simulink model "motorControlSim"  (R2021a)
settings: Solver=VariableStepAuto  StartTime=0.0  StopTime=10  RelTol=1e-3
libraries: fl_lib x9, nesl_utility x9, mcbcontrolslib x8, pid_lib x5, ee_lib x3
settings Model: Creator=Maxim  LastModifiedBy=Max

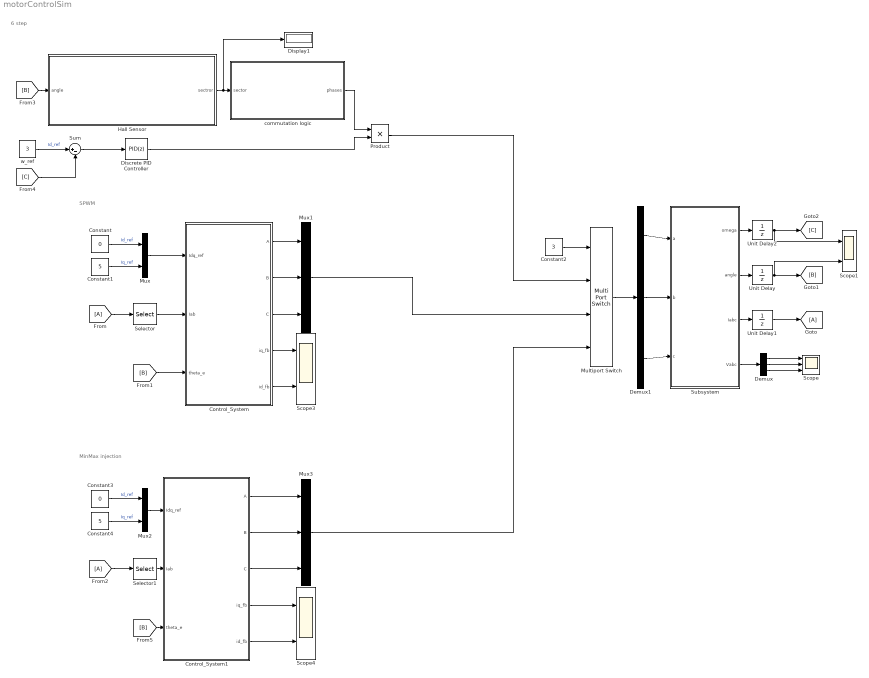
== system motorControlSim ==
  note: 6 step
  note: SPWM
  note: MinMax injection
  Constant : Constant  Value=0  OutDataTypeStr=double
  Constant1 : Constant  Value=5  OutDataTypeStr=double
  Constant2 : Constant  Value=3
  Constant3 : Constant  Value=0  OutDataTypeStr=double
  Constant4 : Constant  Value=5  OutDataTypeStr=double
  Control_System : Subsystem
  Control_System1 : Subsystem
  Demux : Demux  Outputs=3
  Demux1 : Demux  Outputs=3
  Discrete PID Controller : pid_lib/PID Controller  Controller=PID  Form=Parallel  TimeDomain=Discrete-time  UseExternalTs=off  SampleTime=-1  IntegratorMethod=Forward Euler  FilterMethod=Forward Euler  ControllerParametersSource=internal  P=1  I=0.5  D=0  UseFilter=on  N=100  TunerSelectOption=Transfer Function Based (PID Tuner App)  InitialConditionSource=internal  InitialConditionForIntegrator=0  InitialConditionForFilter=0  DifferentiatorICPrevScaledInput=0  ExternalReset=none  TrackingMode=off  Kt=1  LimitOutput=off  SatLimitsSource=internal  UpperSaturationLimit=1  LowerSaturationLimit=0  LinearizeAsGain=off  AntiWindupMode=back-calculation  Kb=1  POutMin=[]  POutMax=[]  IOutMin=[]  IOutMax=[]  DOutMin=[]  DOutMax=[]  NOutMin=[]  NOutMax=[]  SumOutMin=[]  SumOutMax=[]  SaturationOutMin=[]  SaturationOutMax=[]  PParamMin=[]  PParamMax=[]  IParamMin=[]  IParamMax=[]  DParamMin=[]  DParamMax=[]  NParamMin=[]  NParamMax=[]  KbParamMin=[]  KbParamMax=[]  KtParamMin=[]  KtParamMax=[]  KbOutMin=[]  KbOutMax=[]  KtOutMin=[]  KtOutMax=[]  IntegratorOutMin=[]  IntegratorOutMax=[]  FilterOutMin=[]  FilterOutMax=[]  SumI1OutMin=[]  SumI1OutMax=[]  SumI2OutMin=[]  SumI2OutMax=[]  SumI3OutMin=[]  SumI3OutMax=[]  SumI4OutMin=[]  SumI4OutMax=[]  SumDOutMin=[]  SumDOutMax=[]  DifferentiatorOutMin=[]  DifferentiatorOutMax=[]  FilterDiffOutCoefMin=[]  FilterDiffOutCoefMax=[]  ReciprocalOutMin=[]  ReciprocalOutMax=[]  SumDenOutMin=[]  SumDenOutMax=[]  SumNumOutMin=[]  SumNumOutMax=[]  DivideOutMin=[]  DivideOutMax=[]  UdiffTsProdOutMin=[]  UdiffTsProdOutMax=[]  NTsProdOutMin=[]  NTsProdOutMax=[]  UintegralTsProdOutMin=[]  UintegralTsProdOutMax=[]  UngainTsProdOutMin=[]  UngainTsProdOutMax=[]  IntegratorContinuousStateAttributes=''  IntegratorStateMustResolveToSignalObject=off  IntegratorRTWStateStorageClass=Auto  FilterContinuousStateAttributes=''  FilterStateMustResolveToSignalObject=off  FilterRTWStateStorageClass=Auto  ParallelPVariant=InternalParameters  IdealPVariant=Disabled  IVariant=InternalParameters  DVariant=InternalParameters  IntegratorVariant=Discrete  SatVariant=Disabled  AWVariant=Passthrough  PCopyVariant=Disabled  TRVariant=Disabled  FdbkBlocksVariant=Forward  IdealPFdbkVariant=Disabled  SatFdbkVariant=Disabled  DerivativeFilterVariant=ForwardEulerFilter  NVariant=InternalParameters  NCopyVariant=Disabled  FilterICVariant=InternalICsFilter  IntegratorICVariant=InternalICs  ExternalResetVariant=Disabled  TRSumVariant=Passthrough  SumFdbkVariant=Disabled  SumVariant=Sum_PID  TsampFilterVariant=InternalTs  TsampNgainVariant=Passthrough  TsampIntegralVariant=Passthrough  ExternalSaturationOutDataTypeStr=Inherit: Same as second input
  Display1 : Display
  Hall Sensor : Subsystem
  Multiport Switch : MultiPortSwitch
  Mux : Mux  Inputs=2
  Mux1 : Mux  Inputs=3
  Mux2 : Mux  Inputs=2
  Mux3 : Mux  Inputs=3
  Product : Product
  Scope : Scope  NumInputPorts=3
  Scope1 : Scope  NumInputPorts=2
  Scope3 : Scope  NumInputPorts=2
  Scope4 : Scope  NumInputPorts=2
  Selector : Selector  InputPortWidth=3  IndexOptions=Index vector (dialog)  Indices=[1 2]  OutputSizes=1
  Selector1 : Selector  InputPortWidth=3  IndexOptions=Index vector (dialog)  Indices=[1 2]  OutputSizes=1
  Subsystem : Subsystem
  Sum : Sum  Inputs=|+-
  Unit Delay : UnitDelay  SampleTime=-1  HasFrameUpgradeWarning=on
  Unit Delay1 : UnitDelay  SampleTime=-1  HasFrameUpgradeWarning=on
  Unit Delay2 : UnitDelay  SampleTime=-1  HasFrameUpgradeWarning=on
  commutation logic : Subsystem
  w_ref : Constant  Value=3  OutDataTypeStr=double
  wires:
  Selector/1 -> Control_System/2(Iab)
  Constant1/1 -> Mux/2  "Iq_ref"
  Mux/1 -> Control_System/1(Idq_ref)
  Constant/1 -> Mux/1  "Id_ref"
  Subsystem/3(Iabc) -> Unit Delay1/1
  [A] -> Selector/1
  Subsystem/1(omega) -> Unit Delay2/1
  Subsystem/2(angle) -> Unit Delay/1
  [B] -> Control_System/3(theta_e)
  Subsystem/4(Vabc) -> Demux/1
  Demux/1 -> Scope/1
  Demux/2 -> Scope/2
  Demux/3 -> Scope/3
  Unit Delay/1 -> Scope1/2, [B]
  Unit Delay1/1 -> [A]
  Control_System/1(A) -> Mux1/1
  Control_System/2(B) -> Mux1/2
  Control_System/3(C) -> Mux1/3
  Demux1/1 -> Subsystem/1(a)
  Demux1/2 -> Subsystem/2(b)
  Demux1/3 -> Subsystem/3(c)
  Multiport Switch/1 -> Demux1/1
  Mux1/1 -> Multiport Switch/3
  w_ref/1 -> Sum/1  "Id_ref"
  [C] -> Sum/2
  Sum/1 -> Discrete PID Controller/1
  Discrete PID Controller/1 -> Product/2
  Product/1 -> Multiport Switch/2
  Constant2/1 -> Multiport Switch/1
  Unit Delay2/1 -> Scope1/1, [C]
  [B] -> Hall Sensor/1(angle)
  Hall Sensor/1(sectror) -> Display1/1, commutation logic/1(sector)
  commutation logic/1(phases) -> Product/1
  Mux3/1 -> Multiport Switch/4
  Control_System1/2(B) -> Mux3/2
  Control_System1/3(C) -> Mux3/3
  Constant3/1 -> Mux2/1  "Id_ref"
  Mux2/1 -> Control_System1/1(Idq_ref)
  [B] -> Control_System1/3(theta_e)
  Constant4/1 -> Mux2/2  "Iq_ref"
  [A] -> Selector1/1
  Selector1/1 -> Control_System1/2(Iab)
  Control_System/4(iq_fb) -> Scope3/1
  Control_System/5(id_fb) -> Scope3/2
  Control_System1/4(iq_fb) -> Scope4/1
  Control_System1/5(id_fb) -> Scope4/2
  Control_System1/1(A) -> Mux3/1

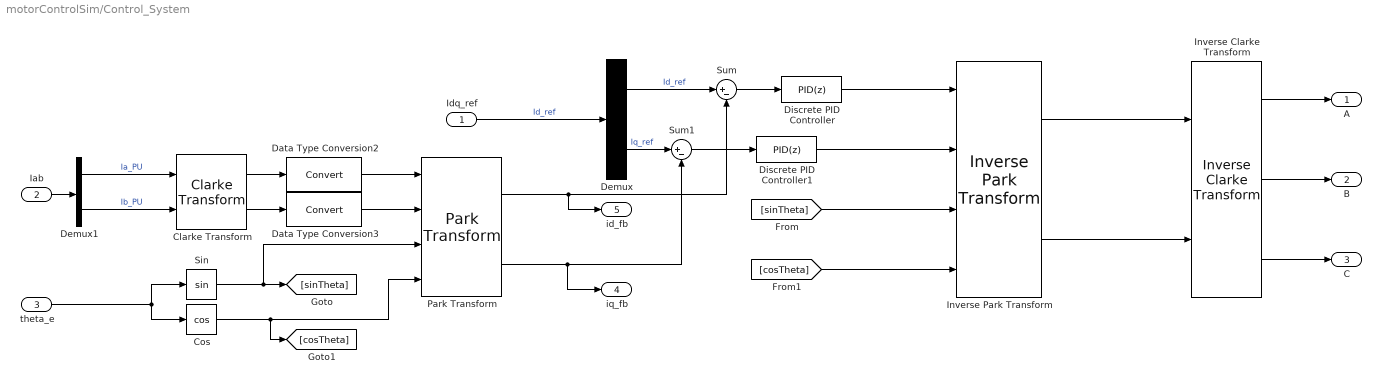
== system motorControlSim/Control_System ==
  Idq_ref : Inport
  Iab : Inport  Port=2
  theta_e : Inport  Port=3
  Clarke Transform : mcbcontrolslib/Clarke Transform  VariantControl=Variant2
  Cos : Trigonometry  Operator=cos
  Data Type Conversion2 : DataTypeConversion
  Data Type Conversion3 : DataTypeConversion
  Demux : Demux  Outputs=2
  Demux1 : Demux  Outputs=2
  Discrete PID Controller : pid_lib/PID Controller  Controller=PID  Form=Parallel  TimeDomain=Discrete-time  UseExternalTs=off  SampleTime=-1  IntegratorMethod=Forward Euler  FilterMethod=Forward Euler  ControllerParametersSource=internal  P=3  I=0.3  D=0  UseFilter=on  N=100  TunerSelectOption=Transfer Function Based (PID Tuner App)  InitialConditionSource=internal  InitialConditionForIntegrator=0  InitialConditionForFilter=0  DifferentiatorICPrevScaledInput=0  ExternalReset=none  TrackingMode=off  Kt=1  LimitOutput=on  SatLimitsSource=internal  UpperSaturationLimit=24  LowerSaturationLimit=-24  LinearizeAsGain=off  AntiWindupMode=back-calculation  Kb=1  POutMin=[]  POutMax=[]  IOutMin=[]  IOutMax=[]  DOutMin=[]  DOutMax=[]  NOutMin=[]  NOutMax=[]  SumOutMin=[]  SumOutMax=[]  SaturationOutMin=[]  SaturationOutMax=[]  PParamMin=[]  PParamMax=[]  IParamMin=[]  IParamMax=[]  DParamMin=[]  DParamMax=[]  NParamMin=[]  NParamMax=[]  KbParamMin=[]  KbParamMax=[]  KtParamMin=[]  KtParamMax=[]  KbOutMin=[]  KbOutMax=[]  KtOutMin=[]  KtOutMax=[]  IntegratorOutMin=[]  IntegratorOutMax=[]  FilterOutMin=[]  FilterOutMax=[]  SumI1OutMin=[]  SumI1OutMax=[]  SumI2OutMin=[]  SumI2OutMax=[]  SumI3OutMin=[]  SumI3OutMax=[]  SumI4OutMin=[]  SumI4OutMax=[]  SumDOutMin=[]  SumDOutMax=[]  DifferentiatorOutMin=[]  DifferentiatorOutMax=[]  FilterDiffOutCoefMin=[]  FilterDiffOutCoefMax=[]  ReciprocalOutMin=[]  ReciprocalOutMax=[]  SumDenOutMin=[]  SumDenOutMax=[]  SumNumOutMin=[]  SumNumOutMax=[]  DivideOutMin=[]  DivideOutMax=[]  UdiffTsProdOutMin=[]  UdiffTsProdOutMax=[]  NTsProdOutMin=[]  NTsProdOutMax=[]  UintegralTsProdOutMin=[]  UintegralTsProdOutMax=[]  UngainTsProdOutMin=[]  UngainTsProdOutMax=[]  IntegratorContinuousStateAttributes=''  IntegratorStateMustResolveToSignalObject=off  IntegratorRTWStateStorageClass=Auto  FilterContinuousStateAttributes=''  FilterStateMustResolveToSignalObject=off  FilterRTWStateStorageClass=Auto  ParallelPVariant=InternalParameters  IdealPVariant=Disabled  IVariant=InternalParameters  DVariant=InternalParameters  IntegratorVariant=Discrete  SatVariant=Enabled  AWVariant=BackCalculation  PCopyVariant=Disabled  TRVariant=Disabled  FdbkBlocksVariant=Forward  IdealPFdbkVariant=Disabled  SatFdbkVariant=Disabled  DerivativeFilterVariant=ForwardEulerFilter  NVariant=InternalParameters  NCopyVariant=Disabled  FilterICVariant=InternalICsFilter  IntegratorICVariant=InternalICs  ExternalResetVariant=Disabled  TRSumVariant=Passthrough  SumFdbkVariant=Disabled  SumVariant=Sum_PID  TsampFilterVariant=InternalTs  TsampNgainVariant=Passthrough  TsampIntegralVariant=Passthrough  ExternalSaturationOutDataTypeStr=Inherit: Same as second input
  Discrete PID Controller1 : pid_lib/PID Controller  Controller=PID  Form=Parallel  TimeDomain=Discrete-time  UseExternalTs=off  SampleTime=-1  IntegratorMethod=Forward Euler  FilterMethod=Forward Euler  ControllerParametersSource=internal  P=3  I=0.3  D=0  UseFilter=on  N=100  TunerSelectOption=Transfer Function Based (PID Tuner App)  InitialConditionSource=internal  InitialConditionForIntegrator=0  InitialConditionForFilter=0  DifferentiatorICPrevScaledInput=0  ExternalReset=none  TrackingMode=off  Kt=1  LimitOutput=on  SatLimitsSource=internal  UpperSaturationLimit=24  LowerSaturationLimit=-24  LinearizeAsGain=off  AntiWindupMode=back-calculation  Kb=1  POutMin=[]  POutMax=[]  IOutMin=[]  IOutMax=[]  DOutMin=[]  DOutMax=[]  NOutMin=[]  NOutMax=[]  SumOutMin=[]  SumOutMax=[]  SaturationOutMin=[]  SaturationOutMax=[]  PParamMin=[]  PParamMax=[]  IParamMin=[]  IParamMax=[]  DParamMin=[]  DParamMax=[]  NParamMin=[]  NParamMax=[]  KbParamMin=[]  KbParamMax=[]  KtParamMin=[]  KtParamMax=[]  KbOutMin=[]  KbOutMax=[]  KtOutMin=[]  KtOutMax=[]  IntegratorOutMin=[]  IntegratorOutMax=[]  FilterOutMin=[]  FilterOutMax=[]  SumI1OutMin=[]  SumI1OutMax=[]  SumI2OutMin=[]  SumI2OutMax=[]  SumI3OutMin=[]  SumI3OutMax=[]  SumI4OutMin=[]  SumI4OutMax=[]  SumDOutMin=[]  SumDOutMax=[]  DifferentiatorOutMin=[]  DifferentiatorOutMax=[]  FilterDiffOutCoefMin=[]  FilterDiffOutCoefMax=[]  ReciprocalOutMin=[]  ReciprocalOutMax=[]  SumDenOutMin=[]  SumDenOutMax=[]  SumNumOutMin=[]  SumNumOutMax=[]  DivideOutMin=[]  DivideOutMax=[]  UdiffTsProdOutMin=[]  UdiffTsProdOutMax=[]  NTsProdOutMin=[]  NTsProdOutMax=[]  UintegralTsProdOutMin=[]  UintegralTsProdOutMax=[]  UngainTsProdOutMin=[]  UngainTsProdOutMax=[]  IntegratorContinuousStateAttributes=''  IntegratorStateMustResolveToSignalObject=off  IntegratorRTWStateStorageClass=Auto  FilterContinuousStateAttributes=''  FilterStateMustResolveToSignalObject=off  FilterRTWStateStorageClass=Auto  ParallelPVariant=InternalParameters  IdealPVariant=Disabled  IVariant=InternalParameters  DVariant=InternalParameters  IntegratorVariant=Discrete  SatVariant=Enabled  AWVariant=BackCalculation  PCopyVariant=Disabled  TRVariant=Disabled  FdbkBlocksVariant=Forward  IdealPFdbkVariant=Disabled  SatFdbkVariant=Disabled  DerivativeFilterVariant=ForwardEulerFilter  NVariant=InternalParameters  NCopyVariant=Disabled  FilterICVariant=InternalICsFilter  IntegratorICVariant=InternalICs  ExternalResetVariant=Disabled  TRSumVariant=Passthrough  SumFdbkVariant=Disabled  SumVariant=Sum_PID  TsampFilterVariant=InternalTs  TsampNgainVariant=Passthrough  TsampIntegralVariant=Passthrough  ExternalSaturationOutDataTypeStr=Inherit: Same as second input
  Inverse Clarke Transform : mcbcontrolslib/Inverse Clarke Transform
      settings: SourceProductBaseCode=MT
  Inverse Park Transform : mcbcontrolslib/Inverse Park Transform  AxisAlignment=D-axis
  Park Transform : mcbcontrolslib/Park Transform  AxisAlignment=D-axis
      settings: SourceProductBaseCode=MT
  Sin : Trigonometry
  Sum : Sum  Inputs=|+-  OutDataTypeStr=Inherit: Same as first input
  Sum1 : Sum  Inputs=|+-  OutDataTypeStr=Inherit: Same as first input
  A : Outport
  B : Outport  Port=2
  C : Outport  Port=3
  iq_fb : Outport  Port=4
  id_fb : Outport  Port=5
  wires:
  Sin/1 -> [sinTheta], Park Transform/3
  Cos/1 -> Park Transform/4, [cosTheta]
  [cosTheta] -> Inverse Park Transform/4
  [sinTheta] -> Inverse Park Transform/3
  Clarke Transform/2 -> Data Type Conversion3/1
  Demux1/1 -> Clarke Transform/1  "Ia_PU"
  Demux1/2 -> Clarke Transform/2  "Ib_PU"
  Iab/1 -> Demux1/1
  Inverse Clarke Transform/1 -> A/1
  Inverse Clarke Transform/2 -> B/1
  Inverse Clarke Transform/3 -> C/1
  Inverse Park Transform/2 -> Inverse Clarke Transform/2
  Inverse Park Transform/1 -> Inverse Clarke Transform/1
  Data Type Conversion2/1 -> Park Transform/1
  Clarke Transform/1 -> Data Type Conversion2/1
  Data Type Conversion3/1 -> Park Transform/2
  theta_e/1 -> Sin/1, Cos/1
  Idq_ref/1 -> Demux/1  "Id_ref"
  Demux/1 -> Sum/1  "Id_ref"
  Demux/2 -> Sum1/1  "Iq_ref"
  Sum/1 -> Discrete PID Controller/1
  Sum1/1 -> Discrete PID Controller1/1
  Park Transform/2 -> iq_fb/1, Sum1/2
  Park Transform/1 -> id_fb/1, Sum/2
  Discrete PID Controller1/1 -> Inverse Park Transform/2
  Discrete PID Controller/1 -> Inverse Park Transform/1

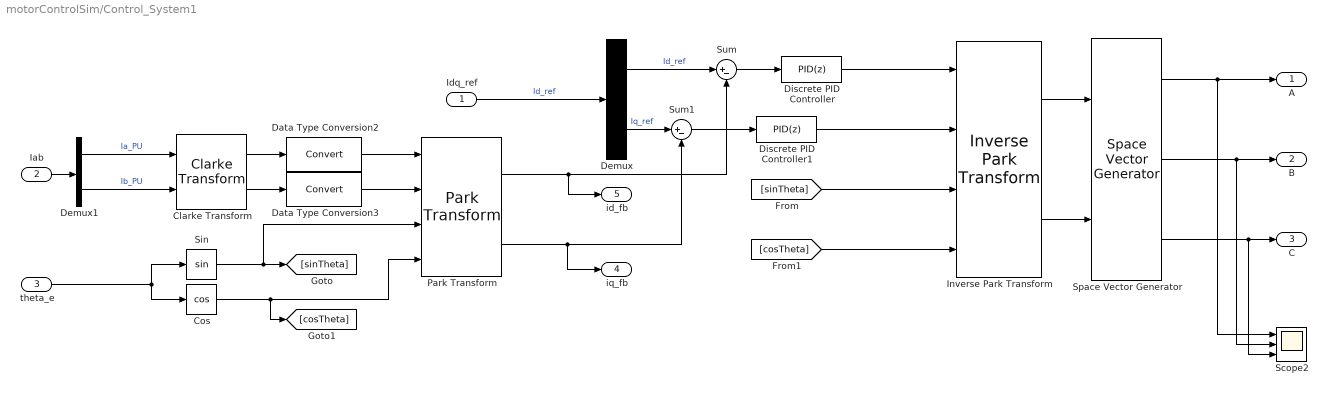
== system motorControlSim/Control_System1 ==
  Idq_ref : Inport
  Iab : Inport  Port=2
  theta_e : Inport  Port=3
  Clarke Transform : mcbcontrolslib/Clarke Transform  VariantControl=Variant2
  Cos : Trigonometry  Operator=cos
  Data Type Conversion2 : DataTypeConversion
  Data Type Conversion3 : DataTypeConversion
  Demux : Demux  Outputs=2
  Demux1 : Demux  Outputs=2
  Discrete PID Controller : pid_lib/PID Controller  Controller=PID  Form=Parallel  TimeDomain=Discrete-time  UseExternalTs=off  SampleTime=2.5e-6  IntegratorMethod=Forward Euler  FilterMethod=Forward Euler  ControllerParametersSource=internal  P=3  I=0.3  D=0  UseFilter=on  N=100  TunerSelectOption=Transfer Function Based (PID Tuner App)  InitialConditionSource=internal  InitialConditionForIntegrator=0  InitialConditionForFilter=0  DifferentiatorICPrevScaledInput=0  ExternalReset=none  TrackingMode=off  Kt=1  LimitOutput=on  SatLimitsSource=internal  UpperSaturationLimit=24  LowerSaturationLimit=-24  LinearizeAsGain=off  AntiWindupMode=back-calculation  Kb=1  POutMin=[]  POutMax=[]  IOutMin=[]  IOutMax=[]  DOutMin=[]  DOutMax=[]  NOutMin=[]  NOutMax=[]  SumOutMin=[]  SumOutMax=[]  SaturationOutMin=[]  SaturationOutMax=[]  PParamMin=[]  PParamMax=[]  IParamMin=[]  IParamMax=[]  DParamMin=[]  DParamMax=[]  NParamMin=[]  NParamMax=[]  KbParamMin=[]  KbParamMax=[]  KtParamMin=[]  KtParamMax=[]  KbOutMin=[]  KbOutMax=[]  KtOutMin=[]  KtOutMax=[]  IntegratorOutMin=[]  IntegratorOutMax=[]  FilterOutMin=[]  FilterOutMax=[]  SumI1OutMin=[]  SumI1OutMax=[]  SumI2OutMin=[]  SumI2OutMax=[]  SumI3OutMin=[]  SumI3OutMax=[]  SumI4OutMin=[]  SumI4OutMax=[]  SumDOutMin=[]  SumDOutMax=[]  DifferentiatorOutMin=[]  DifferentiatorOutMax=[]  FilterDiffOutCoefMin=[]  FilterDiffOutCoefMax=[]  ReciprocalOutMin=[]  ReciprocalOutMax=[]  SumDenOutMin=[]  SumDenOutMax=[]  SumNumOutMin=[]  SumNumOutMax=[]  DivideOutMin=[]  DivideOutMax=[]  UdiffTsProdOutMin=[]  UdiffTsProdOutMax=[]  NTsProdOutMin=[]  NTsProdOutMax=[]  UintegralTsProdOutMin=[]  UintegralTsProdOutMax=[]  UngainTsProdOutMin=[]  UngainTsProdOutMax=[]  IntegratorContinuousStateAttributes=''  IntegratorStateMustResolveToSignalObject=off  IntegratorRTWStateStorageClass=Auto  FilterContinuousStateAttributes=''  FilterStateMustResolveToSignalObject=off  FilterRTWStateStorageClass=Auto  ParallelPVariant=InternalParameters  IdealPVariant=Disabled  IVariant=InternalParameters  DVariant=InternalParameters  IntegratorVariant=Discrete  SatVariant=Enabled  AWVariant=BackCalculation  PCopyVariant=Disabled  TRVariant=Disabled  FdbkBlocksVariant=Forward  IdealPFdbkVariant=Disabled  SatFdbkVariant=Disabled  DerivativeFilterVariant=ForwardEulerFilter  NVariant=InternalParameters  NCopyVariant=Disabled  FilterICVariant=InternalICsFilter  IntegratorICVariant=InternalICs  ExternalResetVariant=Disabled  TRSumVariant=Passthrough  SumFdbkVariant=Disabled  SumVariant=Sum_PID  TsampFilterVariant=InternalTs  TsampNgainVariant=Passthrough  TsampIntegralVariant=Passthrough  ExternalSaturationOutDataTypeStr=Inherit: Same as second input
  Discrete PID Controller1 : pid_lib/PID Controller  Controller=PID  Form=Parallel  TimeDomain=Discrete-time  UseExternalTs=off  SampleTime=2.5e-6  IntegratorMethod=Forward Euler  FilterMethod=Forward Euler  ControllerParametersSource=internal  P=3  I=0.3  D=0  UseFilter=on  N=100  TunerSelectOption=Transfer Function Based (PID Tuner App)  InitialConditionSource=internal  InitialConditionForIntegrator=0  InitialConditionForFilter=0  DifferentiatorICPrevScaledInput=0  ExternalReset=none  TrackingMode=off  Kt=1  LimitOutput=on  SatLimitsSource=internal  UpperSaturationLimit=24  LowerSaturationLimit=-24  LinearizeAsGain=off  AntiWindupMode=back-calculation  Kb=1  POutMin=[]  POutMax=[]  IOutMin=[]  IOutMax=[]  DOutMin=[]  DOutMax=[]  NOutMin=[]  NOutMax=[]  SumOutMin=[]  SumOutMax=[]  SaturationOutMin=[]  SaturationOutMax=[]  PParamMin=[]  PParamMax=[]  IParamMin=[]  IParamMax=[]  DParamMin=[]  DParamMax=[]  NParamMin=[]  NParamMax=[]  KbParamMin=[]  KbParamMax=[]  KtParamMin=[]  KtParamMax=[]  KbOutMin=[]  KbOutMax=[]  KtOutMin=[]  KtOutMax=[]  IntegratorOutMin=[]  IntegratorOutMax=[]  FilterOutMin=[]  FilterOutMax=[]  SumI1OutMin=[]  SumI1OutMax=[]  SumI2OutMin=[]  SumI2OutMax=[]  SumI3OutMin=[]  SumI3OutMax=[]  SumI4OutMin=[]  SumI4OutMax=[]  SumDOutMin=[]  SumDOutMax=[]  DifferentiatorOutMin=[]  DifferentiatorOutMax=[]  FilterDiffOutCoefMin=[]  FilterDiffOutCoefMax=[]  ReciprocalOutMin=[]  ReciprocalOutMax=[]  SumDenOutMin=[]  SumDenOutMax=[]  SumNumOutMin=[]  SumNumOutMax=[]  DivideOutMin=[]  DivideOutMax=[]  UdiffTsProdOutMin=[]  UdiffTsProdOutMax=[]  NTsProdOutMin=[]  NTsProdOutMax=[]  UintegralTsProdOutMin=[]  UintegralTsProdOutMax=[]  UngainTsProdOutMin=[]  UngainTsProdOutMax=[]  IntegratorContinuousStateAttributes=''  IntegratorStateMustResolveToSignalObject=off  IntegratorRTWStateStorageClass=Auto  FilterContinuousStateAttributes=''  FilterStateMustResolveToSignalObject=off  FilterRTWStateStorageClass=Auto  ParallelPVariant=InternalParameters  IdealPVariant=Disabled  IVariant=InternalParameters  DVariant=InternalParameters  IntegratorVariant=Discrete  SatVariant=Enabled  AWVariant=BackCalculation  PCopyVariant=Disabled  TRVariant=Disabled  FdbkBlocksVariant=Forward  IdealPFdbkVariant=Disabled  SatFdbkVariant=Disabled  DerivativeFilterVariant=ForwardEulerFilter  NVariant=InternalParameters  NCopyVariant=Disabled  FilterICVariant=InternalICsFilter  IntegratorICVariant=InternalICs  ExternalResetVariant=Disabled  TRSumVariant=Passthrough  SumFdbkVariant=Disabled  SumVariant=Sum_PID  TsampFilterVariant=InternalTs  TsampNgainVariant=Passthrough  TsampIntegralVariant=Passthrough  ExternalSaturationOutDataTypeStr=Inherit: Same as second input
  Inverse Park Transform : mcbcontrolslib/Inverse Park Transform  AxisAlignment=D-axis
  Park Transform : mcbcontrolslib/Park Transform  AxisAlignment=D-axis
      settings: SourceProductBaseCode=MT
  Scope2 : Scope  NumInputPorts=3
  Sin : Trigonometry
  Space Vector Generator : mcbcontrolslib/Space Vector Generator
      settings: SourceProductBaseCode=MT
  Sum : Sum  Inputs=|+-  OutDataTypeStr=Inherit: Same as first input
  Sum1 : Sum  Inputs=|+-  OutDataTypeStr=Inherit: Same as first input
  A : Outport
  B : Outport  Port=2
  C : Outport  Port=3
  iq_fb : Outport  Port=4
  id_fb : Outport  Port=5
  wires:
  Sin/1 -> [sinTheta], Park Transform/3
  Cos/1 -> Park Transform/4, [cosTheta]
  [cosTheta] -> Inverse Park Transform/4
  [sinTheta] -> Inverse Park Transform/3
  Clarke Transform/2 -> Data Type Conversion3/1
  Demux1/1 -> Clarke Transform/1  "Ia_PU"
  Demux1/2 -> Clarke Transform/2  "Ib_PU"
  Iab/1 -> Demux1/1
  Inverse Park Transform/2 -> Space Vector Generator/2
  Inverse Park Transform/1 -> Space Vector Generator/1
  Data Type Conversion2/1 -> Park Transform/1
  Clarke Transform/1 -> Data Type Conversion2/1
  Data Type Conversion3/1 -> Park Transform/2
  theta_e/1 -> Sin/1, Cos/1
  Idq_ref/1 -> Demux/1  "Id_ref"
  Demux/1 -> Sum/1  "Id_ref"
  Demux/2 -> Sum1/1  "Iq_ref"
  Sum/1 -> Discrete PID Controller/1
  Sum1/1 -> Discrete PID Controller1/1
  Discrete PID Controller1/1 -> Inverse Park Transform/2
  Discrete PID Controller/1 -> Inverse Park Transform/1
  Park Transform/1 -> id_fb/1, Sum/2
  Park Transform/2 -> iq_fb/1, Sum1/2
  Space Vector Generator/1 -> Scope2/1, A/1
  Space Vector Generator/2 -> Scope2/2, B/1
  Space Vector Generator/3 -> Scope2/3, C/1

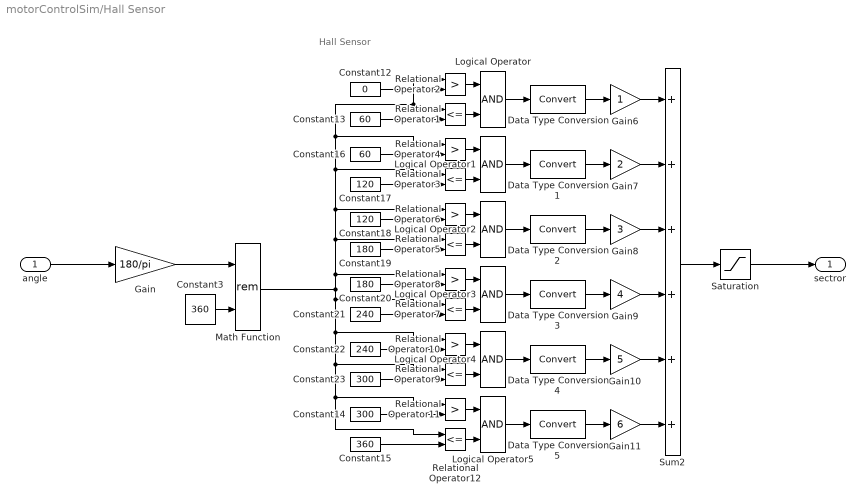
== system motorControlSim/Hall Sensor ==
  note: Hall Sensor
  angle : Inport
  Constant12 : Constant  Value=0
  Constant13 : Constant  Value=60
  Constant14 : Constant  Value=300
  Constant15 : Constant  Value=360
  Constant16 : Constant  Value=60
  Constant17 : Constant  Value=120
  Constant18 : Constant  Value=120
  Constant19 : Constant  Value=180
  Constant20 : Constant  Value=180
  Constant21 : Constant  Value=240
  Constant22 : Constant  Value=240
  Constant23 : Constant  Value=300
  Constant3 : Constant  Value=360
  Data Type Conversion{,1..5} (6 alike) : DataTypeConversion  SaturateOnIntegerOverflow=on  RndMeth=Zero
  Gain : Gain  Gain=180/pi
  Gain10 : Gain  Gain=5  SaturateOnIntegerOverflow=on  OutDataTypeStr=Inherit: Same as input  ParamDataTypeStr=Inherit: Same as input
  Gain11 : Gain  Gain=6  SaturateOnIntegerOverflow=on  OutDataTypeStr=Inherit: Same as input  ParamDataTypeStr=Inherit: Same as input
  Gain6 : Gain  SaturateOnIntegerOverflow=on  OutDataTypeStr=Inherit: Same as input  ParamDataTypeStr=Inherit: Same as input
  Gain7 : Gain  Gain=2  SaturateOnIntegerOverflow=on  OutDataTypeStr=Inherit: Same as input  ParamDataTypeStr=Inherit: Same as input
  Gain8 : Gain  Gain=3  SaturateOnIntegerOverflow=on  OutDataTypeStr=Inherit: Same as input  ParamDataTypeStr=Inherit: Same as input
  Gain9 : Gain  Gain=4  SaturateOnIntegerOverflow=on  OutDataTypeStr=Inherit: Same as input  ParamDataTypeStr=Inherit: Same as input
  Logical Operator{,1..5} (6 alike) : Logic
  Math Function : Math  Operator=rem  SignedPower=on  SaturateOnIntegerOverflow=on
  Relational Operator{1,3,5,7,9,12} (6 alike) : RelationalOperator  Operator=<=  RndMeth=Nearest  InputSameDT=on
  Relational Operator{2,4,6,8,10..11} (6 alike) : RelationalOperator  Operator=>  RndMeth=Nearest  InputSameDT=on
  Saturation : Saturate  UpperLimit=6  LowerLimit=1
  Sum2 : Sum  Inputs=++++++  InputSameDT=on  SaturateOnIntegerOverflow=on  OutDataTypeStr=Inherit: Same as first input
  sectror : Outport
  wires:
  Data Type Conversion1/1 -> Gain7/1
  Relational Operator2/1 -> Logical Operator/1
  Relational Operator9/1 -> Logical Operator4/2
  Constant12/1 -> Relational Operator2/2
  Constant18/1 -> Relational Operator6/2
  Data Type Conversion/1 -> Gain6/1
  Logical Operator3/1 -> Data Type Conversion3/1
  Saturation/1 -> sectror/1
  Data Type Conversion3/1 -> Gain9/1
  Gain11/1 -> Sum2/6
  Relational Operator3/1 -> Logical Operator1/2
  Constant16/1 -> Relational Operator4/2
  angle/1 -> Gain/1
  Relational Operator6/1 -> Logical Operator2/1
  Relational Operator8/1 -> Logical Operator3/1
  Constant23/1 -> Relational Operator9/2
  Gain10/1 -> Sum2/5
  Constant17/1 -> Relational Operator3/2
  Relational Operator1/1 -> Logical Operator/2
  Relational Operator10/1 -> Logical Operator4/1
  Logical Operator2/1 -> Data Type Conversion2/1
  Logical Operator1/1 -> Data Type Conversion1/1
  Logical Operator5/1 -> Data Type Conversion5/1
  Gain9/1 -> Sum2/4
  Constant13/1 -> Relational Operator1/2
  Relational Operator4/1 -> Logical Operator1/1
  Relational Operator12/1 -> Logical Operator5/2
  Constant20/1 -> Relational Operator8/2
  Sum2/1 -> Saturation/1
  Gain7/1 -> Sum2/2
  Relational Operator5/1 -> Logical Operator2/2
  Constant22/1 -> Relational Operator10/2
  Relational Operator11/1 -> Logical Operator5/1
  Data Type Conversion2/1 -> Gain8/1
  Constant15/1 -> Relational Operator12/2
  Gain8/1 -> Sum2/3
  Gain6/1 -> Sum2/1
  Logical Operator4/1 -> Data Type Conversion4/1
  Constant14/1 -> Relational Operator11/2
  Constant19/1 -> Relational Operator5/2
  Constant21/1 -> Relational Operator7/2
  Relational Operator7/1 -> Logical Operator3/2
  Logical Operator/1 -> Data Type Conversion/1
  Data Type Conversion5/1 -> Gain11/1
  Data Type Conversion4/1 -> Gain10/1
  Math Function/1 -> Relational Operator2/1, Relational Operator1/1, Relational Operator4/1, Relational Operator3/1, Relational Operator6/1, Relational Operator5/1, Relational Operator8/1, Relational Operator12/1, Relational Operator11/1, Relational Operator9/1, Relational Operator10/1, Relational Operator7/1
  Constant3/1 -> Math Function/2
  Gain/1 -> Math Function/1

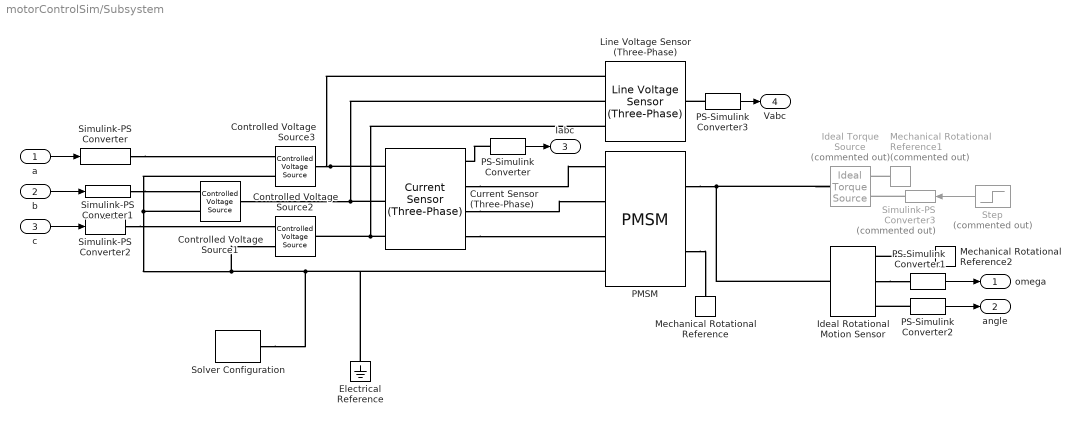
== system motorControlSim/Subsystem ==
  a : Inport
  b : Inport  Port=2
  c : Inport  Port=3
  Controlled Voltage Source1 : fl_lib/Electrical/Electrical Sources/Controlled Voltage Source
  Controlled Voltage Source2 : fl_lib/Electrical/Electrical Sources/Controlled Voltage Source
  Controlled Voltage Source3 : fl_lib/Electrical/Electrical Sources/Controlled Voltage Source
  Current Sensor (Three-Phase) : ee_lib/Sensors & Transducers/Current Sensor (Three-Phase)
      settings: InternalSimscapePortConfiguration="{\"Bottom\":[],\"Left\":[{\"id\":\"a1\",\"label\":\"a1\",\"type\":\"foundation.electrical.electrical\"},{\"id\":\"b1\",\"label\":\"b1\",\"type\":\"foundation.electrical.electrical\"},{\"id\":\"c1\",\"label\":\"c1\",\"type\":\"foundation.electrical.electrical\"}],\"Right\":[{\"id\":\"I_output\",\"label\":\"I\",\"type\":\"output\"},{\"id\":\"a2\",\"label\":\"a2\",\"type\":\"foundation.electrical.electrical\"},{\"id\":\"b2\",\"label\":\"b2\",\"type\":\"foundation.electrical.electrical\"},{\"id\":\"c2\",\"label\":\"c2\",\"type\":\"foundation.electrical.electrical\"}],\"Top\":[]}"
  Electrical Reference : fl_lib/Electrical/Electrical Elements/Electrical Reference
  Ideal Rotational Motion Sensor : fl_lib/Mechanical/Mechanical Sensors/Ideal Rotational Motion Sensor  wrap_angle=simscape.enum.onoff.off  offset=0 rad
  Ideal Torque Source : fl_lib/Mechanical/Mechanical Sources/Ideal Torque Source  Commented=on
  Line Voltage Sensor (Three-Phase) : ee_lib/Sensors & Transducers/Line Voltage Sensor (Three-Phase)
      settings: SourceProductBaseCode=PS  InternalSimscapePortConfiguration="{\"Bottom\":[],\"Left\":[{\"id\":\"a\",\"label\":\"a\",\"type\":\"foundation.electrical.electrical\"},{\"id\":\"b\",\"label\":\"b\",\"type\":\"foundation.electrical.electrical\"},{\"id\":\"c\",\"label\":\"c\",\"type\":\"foundation.electrical.electrical\"}],\"Right\":[{\"id\":\"V_output\",\"label\":\"V\",\"type\":\"output\"}],\"Top\":[]}"
  Mechanical Rotational Reference : fl_lib/Mechanical/Rotational Elements/Mechanical Rotational Reference
  Mechanical Rotational Reference1 : fl_lib/Mechanical/Rotational Elements/Mechanical Rotational Reference  Commented=on
  Mechanical Rotational Reference2 : fl_lib/Mechanical/Rotational Elements/Mechanical Rotational Reference
  PMSM : ee_lib/Electromechanical/Permanent Magnet/PMSM  winding_type=ee.enum.statorconnection.wye  machine_param=ee.enum.pmsm.parameterization.constant  nPolePairs=1  pmflux_param=ee.enum.pmflux.fluxlinkage  pm_flux_linkage=0.03 Wb  torque_constant=0.18 N*m/A  back_emf_constant=0.18 V/(rad/s)  stator_param=ee.enum.statorparam.LdLqL0  Ld=2.5 mH  Lq=2.5 mH  idVec=[-200, 0, 200] A  iqVec=[-200, 0, 200] A  LdMatrix=0.0002 * ones(3, 3) H  LqMatrix=0.0002 * ones(3, 3) H  PmMatrix=0.1 * ones(3, 3) Wb  ktMatrix=0.18 * ones(3, 3) N*m/A  keMatrix=0.18 * ones(3, 3) V/(rad/s)  L0=2.5 mH  Ls=0.0002 H  Lm=-0.00002 H  Ms=0.00002 H  Rs=0.36 Ohm  zero_sequence=ee.enum.park.zerosequence.include  J=0.01 kg*m^2  lam=0 N*m/(rad/s)  axes_param=ee.enum.rotorangle.daxis  i_d_specify=off  i_d_priority=None  i_d=0 A  i_d_nominal_specify=off  i_d_nominal_unit=A  i_d_nominal_value=1  i_q_specify=off  i_q_priority=None  i_q=0 A  i_q_nominal_specify=off  i_q_nominal_unit=A  i_q_nominal_value=1  torque_specify=off  torque_priority=None  torque=0 N*m  torque_nominal_specify=off  torque_nominal_unit=N*m  torque_nominal_value=1  angular_velocity_specify=off  angular_velocity_priority=High  angular_velocity=0 rpm  angular_velocity_nominal_specify=off  angular_velocity_nominal_unit=rpm  angular_velocity_nominal_value=1  angular_position_specify=off  angular_position_priority=High  angular_position=0 deg  angular_position_nominal_specify=off  angular_position_nominal_unit=deg  angular_position_nominal_value=1  loss_param=ee.enum.ironloss.none  losses_oc=[0, 0, 0] W  losses_sc=[0, 0, 0] W  f_losses=60 Hz  Isc_losses=95 A  Tmeas=298.15 K  alpha=3.93e-3 1/K  alpha_flux=-0.001 1/K  stator_thermal_mass=100 J/K  rotor_thermal_mass=200 J/K  Rm_percent_rotor=90  Rd_percent_rotor=30  temperatureA_specify=off  temperatureA_priority=High  temperatureA=25 degC  temperatureA_nominal_specify=off  temperatureA_nominal_unit=degC  temperatureA_nominal_value=1  temperatureB_specify=off  temperatureB_priority=High  temperatureB=25 degC  temperatureB_nominal_specify=off  temperatureB_nominal_unit=degC  temperatureB_nominal_value=1  temperatureC_specify=off  temperatureC_priority=High  temperatureC=25 degC  temperatureC_nominal_specify=off  temperatureC_nominal_unit=degC  temperatureC_nominal_value=1  temperatureR_specify=off  temperatureR_priority=High  temperatureR=25 degC  temperatureR_nominal_specify=off  temperatureR_nominal_unit=degC  temperatureR_nominal_value=1
      settings: InternalSimscapePortConfiguration="{\"Bottom\":[],\"Left\":[{\"id\":\"a\",\"label\":\"a\",\"type\":\"foundation.electrical.electrical\"},{\"id\":\"b\",\"label\":\"b\",\"type\":\"foundation.electrical.electrical\"},{\"id\":\"c\",\"label\":\"c\",\"type\":\"foundation.electrical.electrical\"},{\"id\":\"n\",\"label\":\"n\",\"type\":\"foundation.electrical.electrical\"}],\"Right\":[{\"id\":\"R\",\"label\":\"R\",\"type\":\"foundation.mechanical.rotational.rotational\"},{\"id\":\"C\",\"label\":\"C\",\"type\":\"foundation.mechanical.rotational.rotational\"}],\"Top\":[]}"
  PS-Simulink Converter{,1..3} (4 alike) : nesl_utility/PS-Simulink Converter  PhysicalDomain=network_engine_domain  SubClassName=ps_output  LeftPortType=input  RightPortType=output  PseudoPeriodic=off  Frequencies=[]  Unit=inherit  AffineConversion=off
      settings: SourceProductBaseCode=PW,SS
  Simulink-PS Converter : nesl_utility/Simulink-PS Converter  PhysicalDomain=network_engine_domain  SubClassName=ps_input  LeftPortType=input  RightPortType=output  PseudoPeriodic=off  Frequencies=[]  NoiseDistribution=none  NoiseParameters=[]  Unit=1  AffineConversion=off  FilteringAndDerivatives=provide  SimscapeFilterOrder=1  InputFilterTimeConstant=0.001  UdotUserProvided=0
      settings: SourceProductBaseCode=PW,SS
  Simulink-PS Converter1 : nesl_utility/Simulink-PS Converter  PhysicalDomain=network_engine_domain  SubClassName=ps_input  LeftPortType=input  RightPortType=output  PseudoPeriodic=off  Frequencies=[]  NoiseDistribution=none  NoiseParameters=[]  Unit=1  AffineConversion=off  FilteringAndDerivatives=provide  SimscapeFilterOrder=1  InputFilterTimeConstant=0.001  UdotUserProvided=0
      settings: SourceProductBaseCode=PW,SS
  Simulink-PS Converter2 : nesl_utility/Simulink-PS Converter  PhysicalDomain=network_engine_domain  SubClassName=ps_input  LeftPortType=input  RightPortType=output  PseudoPeriodic=off  Frequencies=[]  NoiseDistribution=none  NoiseParameters=[]  Unit=1  AffineConversion=off  FilteringAndDerivatives=provide  SimscapeFilterOrder=1  InputFilterTimeConstant=0.001  UdotUserProvided=0
      settings: SourceProductBaseCode=PW,SS
  Simulink-PS Converter3 : nesl_utility/Simulink-PS Converter  Commented=on  PhysicalDomain=network_engine_domain  SubClassName=ps_input  LeftPortType=input  RightPortType=output  PseudoPeriodic=off  Frequencies=[]  NoiseDistribution=none  NoiseParameters=[]  Unit=1  AffineConversion=off  FilteringAndDerivatives=provide  SimscapeFilterOrder=1  InputFilterTimeConstant=0.001  UdotUserProvided=0
      settings: SourceProductBaseCode=PW,SS
  Solver Configuration : nesl_utility/Solver Configuration  PhysicalDomain=network_engine_domain  SubClassName=solver  LeftPortType=input  RightPortType=generic  Tones=[]  Harmonics=[]  SimulateNoise=off  Profile=off  UseLocalSampling=off  EnableSwitchedLinearOptims=on  FrequencyDomain=off  UseCCode=off  RelTol=0.001  AbsTol=1e-06  MinStep=1e-09  ToWorkspace=off  RevertToSquareIcSolve=off  NumHomotopyIterations=100  PhasorMode=off  PhasorModeNumHarmonics=1  DoDC=off  ResidualTolerance=1e-09  UseLocalSolver=on  LocalSolverChoice=NE_PARTITIONING_ADVANCER  LocalSolverSampleTime=2.5e-6  DoFixedCost=on  MaxNonlinIter=3  MaxModeIter=2  ComputeImpulses=off  ImpulseIterations=2  LinearAlgebra=auto  EquationFormulation=NE_TIME_EF  DelaysMemoryBudget=1024  AutomaticFiltering=on  FilteringTimeConstant=0.001  PartitionStorageMethod=AS_NEEDED  PartitionMemoryBudget=1024  PartitionMethod=ROBUST
      settings: SourceProductBaseCode=PW,SS
  Step : Step  Commented=on  Time=0  After=0  SampleTime=0
  omega : Outport
  angle : Outport  Port=2
  Iabc : Outport  Port=3
  Vabc : Outport  Port=4
  wires:
  c/1 -> Simulink-PS Converter2/1
  b/1 -> Simulink-PS Converter1/1
  a/1 -> Simulink-PS Converter/1
  Step/1 -> Simulink-PS Converter3/1
  PS-Simulink Converter1/1 -> omega/1
  PS-Simulink Converter2/1 -> angle/1
  PS-Simulink Converter/1 -> Iabc/1
  PS-Simulink Converter3/1 -> Vabc/1
  connections:
  Controlled Voltage Source3/LConn1 -- Current Sensor (Three-Phase)/LConn1 -- Line Voltage Sensor (Three-Phase)/LConn3
  Controlled Voltage Source1/LConn1 -- Current Sensor (Three-Phase)/LConn2 -- Line Voltage Sensor (Three-Phase)/LConn2
  Controlled Voltage Source1/RConn2 -- Controlled Voltage Source3/RConn2 -- Controlled Voltage Source2/RConn2 -- Solver Configuration/RConn1 -- PMSM/LConn4 -- Electrical Reference/LConn1
  Simulink-PS Converter/RConn1 -- Controlled Voltage Source3/RConn1
  Simulink-PS Converter1/RConn1 -- Controlled Voltage Source1/RConn1
  Simulink-PS Converter2/RConn1 -- Controlled Voltage Source2/RConn1
  PMSM/RConn2 -- Mechanical Rotational Reference/LConn1
  Ideal Rotational Motion Sensor/LConn1 -- Ideal Torque Source/LConn1 -- PMSM/RConn1
  Mechanical Rotational Reference1/LConn1 -- Ideal Torque Source/RConn2
  Mechanical Rotational Reference2/LConn1 -- Ideal Rotational Motion Sensor/RConn1
  Simulink-PS Converter3/RConn1 -- Ideal Torque Source/RConn1
  Ideal Rotational Motion Sensor/RConn2 -- PS-Simulink Converter1/LConn1
  PS-Simulink Converter2/LConn1 -- Ideal Rotational Motion Sensor/RConn3
  Current Sensor (Three-Phase)/LConn3 -- Line Voltage Sensor (Three-Phase)/LConn1 -- Controlled Voltage Source2/LConn1
  Current Sensor (Three-Phase)/RConn4 -- PMSM/LConn3
  Current Sensor (Three-Phase)/RConn2 -- PMSM/LConn1
  Current Sensor (Three-Phase)/RConn3 -- PMSM/LConn2
  PS-Simulink Converter/LConn1 -- Current Sensor (Three-Phase)/RConn1
  PS-Simulink Converter3/LConn1 -- Line Voltage Sensor (Three-Phase)/RConn1

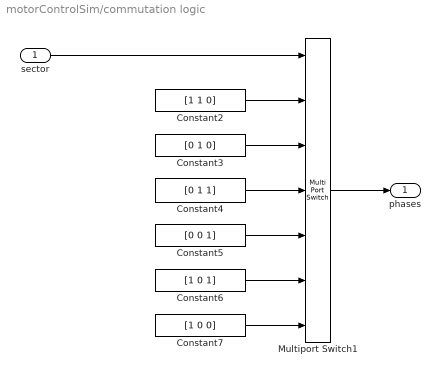
== system motorControlSim/commutation logic ==
  sector : Inport
  Constant2 : Constant  Value=[1 1 0]
  Constant3 : Constant  Value=[0 1 0]
  Constant4 : Constant  Value=[0 1 1]
  Constant5 : Constant  Value=[0 0 1]
  Constant6 : Constant  Value=[1 0 1]
  Constant7 : Constant  Value=[1 0 0]
  Multiport Switch1 : MultiPortSwitch  Inputs=6
  phases : Outport
  wires:
  Constant3/1 -> Multiport Switch1/3
  Constant4/1 -> Multiport Switch1/4
  Constant5/1 -> Multiport Switch1/5
  Constant7/1 -> Multiport Switch1/7
  Constant6/1 -> Multiport Switch1/6
  sector/1 -> Multiport Switch1/1
  Constant2/1 -> Multiport Switch1/2
  Multiport Switch1/1 -> phases/1
